simulink model "MPC_framework"  (Simulink 6.4)
settings: Solver=FixedStepDiscrete  StartTime=0.0  StopTime=10.0  FixedStep=0.01  RelTol=1e-3
PreLoadFcn:
  | RTWConfigurationCB('preloadfcn', bdroot);
InitFcn:
  | % START RTW CONFIGURATION CODE %
  | RTWConfigurationCB('rtw_target_initfcn',gcs);
  | % END RTW CONFIGURATION CODE %
values from neighbouring files (symbols this model uses):
  a1 = 1000    [param_list.m]
  a2 = 750    [param_list.m]
  increments_per_half_turn = uint32(hex2dec('400000'))    [param_list.m]
  init_1_message = uint8(1)    [param-list.m]    (also in param_list.m)
  init_2_message = uint8(2)    [param-list.m]    (also in param_list.m)
  init_ack_async_message = uint8(21)    [param-list.m]    (also in param_list.m)
  init_ack_sync_message = uint8(20)    [param-list.m]    (also in param_list.m)
  motor_negative_value = DA_max * 0.4    [param_list.m]
  motor_positive_value = DA_max * 0.6    [param_list.m]
  motor_stopped_value = DA_max / 2    [param_list.m]
libraries: canblocks x16, mpc555toucan x16, simulink x6, mpc555drivers x1
settings Model: LastModifiedBy=Developer  ProdHWDeviceType=Motorola PowerPC
settings OptimizationCC: OptimizeModelRefInitCode=on  LifeSpan=1
settings HardwareCC: ProdIntDivRoundTo=Zero  ProdEndianess=BigEndian  ProdHWDeviceType=Motorola PowerPC
settings RTWCC: SystemTargetFile=mpc555rt.tlc  TemplateMakefile=mpc555rt.tmf  Description=Embedded Target for Motorola MPC555 (real-time target)  ProcessScript=mpc555rt_make_rtw_hook
settings CodeAppCC: IgnoreCustomStorageClasses=off
settings STFCustomTargetCC: TargetFcnLib=codewarrior_tfl_tmw.mat  TargetLibSuffix=.a  TargetPreCompLibLocation=C:\MATLAB\R2006a\toolbox\rtw\targets\mpc555dk\drivers\lib\CODE_WARRIOR  GenFloatMathFcnCalls=ISO_C  CombineOutputUpdateFcns=on  IncludeERTFirstTime=on  ERTCustomFileBanners=on  SupportContinuousTime=off  SupportNonInlinedSFcns=off  SystemTargetFile=mpc555rt.tlc
settings ERTTargetCC: TargetFcnLib=codewarrior_tfl_tmw.mat  TargetPreCompLibLocation=C:\MATLAB\R2006a\toolbox\rtw\targets\mpc555dk\drivers\lib\CODE_WARRIOR  GenFloatMathFcnCalls=ISO_C  IncludeERTFirstTime=on  ERTFirstTimeCompliant=off  InlinedParameterPlacement=NonHierarchical  ERTCustomFileTemplate=example_file_process.tlc  InitialValueSource=Model
settings CustomProperty: DataType=RTWOptions_EnumType__toolbox_rtw_targets_mpc555dk_mpc555dk_mpc555rt_MPC555_OPTIMIZATION_SWITCH  Value=speed
settings EnumStrPairs: String=speed

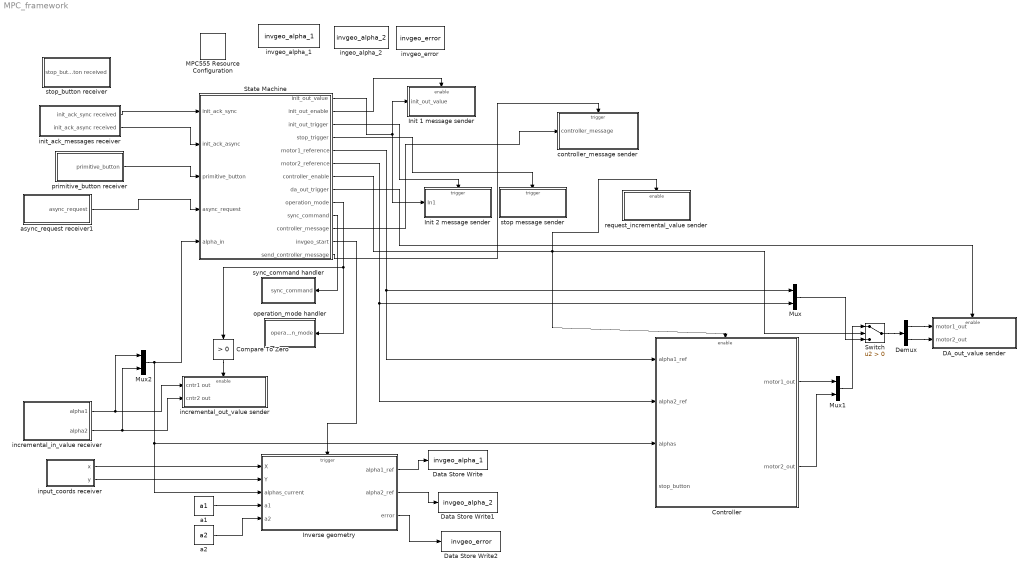
== system MPC_framework ==
  Compare To Zero : simulink/Logic and Bit Operations/Compare To Zero  Orientation=down  SystemSampleTime=-1  relop=>  LogicOutDataTypeMode=uint8  ZeroCross=off
  Controller : Subsystem
  DA_out_value sender : Subsystem  TreatAsAtomicUnit=on
  Data Store Write : DataStoreWrite  DataStoreName=invgeo_alpha_1  SampleTime=-1
  Data Store Write1 : DataStoreWrite  DataStoreName=invgeo_alpha_2  SampleTime=-1
  Data Store Write2 : DataStoreWrite  DataStoreName=invgeo_error  SampleTime=-1
  Demux : Demux  Outputs=2
  Init 1 message sender : Subsystem  TreatAsAtomicUnit=on
  Init 2 message sender : Subsystem  TreatAsAtomicUnit=on
  Inverse geometry : Subsystem  TreatAsAtomicUnit=on
  MPC555 Resource Configuration : mpc555drivers/MPC555 Resource Configuration  Tag=RTW CONFIGURATION BLOCK  Priority=-100000  SystemSampleTime=-1  oldParentName=MPC_framework  oldBlockName=|
      | MPC_framework/MPC555
      | Resource
      | Configuration
  Mux : Mux  Inputs=2
  Mux1 : Mux  Inputs=2
  Mux2 : Mux  Inputs=2
  State Machine : Stateflow chart
  Switch : Switch  Criteria=u2 > Threshold
  a1 : Constant  Value=a1  OutDataType=sfix(16)  ConRadixGroup=Use specified scaling  OutScaling=2^0  SampleTime=inf  FramePeriod=inf
  a2 : Constant  Value=a2  OutDataType=sfix(16)  ConRadixGroup=Use specified scaling  OutScaling=2^0  SampleTime=inf  FramePeriod=inf
  async_request receiver1 : Subsystem
  controller_message sender : Subsystem  TreatAsAtomicUnit=on
  incremental_in_value receiver : Subsystem
  incremental_out_value sender : Subsystem  TreatAsAtomicUnit=on
  ingeo_alpha_2 : DataStoreMemory  DataStoreName=invgeo_alpha_2  ReadBeforeWriteMsg=error  WriteAfterWriteMsg=error  WriteAfterReadMsg=error  InitialValue=0  DataType=double
  init_ack_messages receiver : Subsystem
  input_coords receiver : Subsystem
  invgeo_alpha_1 : DataStoreMemory  DataStoreName=invgeo_alpha_1  ReadBeforeWriteMsg=error  WriteAfterWriteMsg=error  WriteAfterReadMsg=error  InitialValue=0  DataType=double
  invgeo_error : DataStoreMemory  DataStoreName=invgeo_error  ReadBeforeWriteMsg=error  WriteAfterWriteMsg=error  WriteAfterReadMsg=error  InitialValue=0  DataType=uint8
  operation_mode handler : Subsystem  Orientation=left
  primitive_button receiver : Subsystem
  request_incremental_value sender : Subsystem  TreatAsAtomicUnit=on
  stop message sender : Subsystem  TreatAsAtomicUnit=on
  stop_button receiver : Subsystem
  sync_command handler : Subsystem  Orientation=left
  wires:
  State Machine/1(init_out_value) -> Init 2 message sender/1(In1), Init 1 message sender/1(init_out_value)
  State Machine/2(init_out_enable) -> Init 1 message sender/Enable
  init_ack_messages receiver/1(init_ack_sync received) -> State Machine/1(init_ack_sync)
  init_ack_messages receiver/2(init_ack_async received) -> State Machine/2(init_ack_async)
  State Machine/3(init_out_trigger) -> Init 2 message sender/Trigger
  State Machine/4(stop_trigger) -> stop message sender/Trigger
  primitive_button receiver/1(primitive_button) -> State Machine/3(primitive_button)
  State Machine/7(controller_enable) -> Switch/2, request_incremental_value sender/Enable, Controller/Enable
  State Machine/5(motor1_reference) -> Controller/1(alpha1_ref), Mux/1
  State Machine/6(motor2_reference) -> Controller/2(alpha2_ref), Mux/2
  incremental_in_value receiver/2(alpha2) -> incremental_out_value sender/2(cntr2 out), Mux2/2
  Controller/1(motor1_out) -> Mux1/1
  Controller/2(motor2_out) -> Mux1/2
  Mux1/1 -> Switch/1
  Mux/1 -> Switch/3
  Switch/1 -> Demux/1
  Demux/1 -> DA_out_value sender/1(motor1_out)
  Demux/2 -> DA_out_value sender/2(motor2_out)
  State Machine/8(da_out_trigger) -> DA_out_value sender/Enable
  State Machine/9(operation_mode) -> Compare To Zero/1, operation_mode handler/1(operation_mode)
  async_request receiver1/1(async_request) -> State Machine/4(async_request)
  Compare To Zero/1 -> incremental_out_value sender/Enable
  State Machine/10(sync_command) -> sync_command handler/1(sync_command)
  incremental_in_value receiver/1(alpha1) -> incremental_out_value sender/1(cntr1 out), Mux2/1
  Mux2/1 -> State Machine/5(alpha_in), Controller/3(alphas), Inverse geometry/3(alphas_current)
  a1/1 -> Inverse geometry/4(a1)
  a2/1 -> Inverse geometry/5(a2)
  State Machine/12(invgeo_start) -> Inverse geometry/Trigger
  State Machine/11(controller_message) -> controller_message sender/1(controller_message)
  State Machine/13(send_controller_message) -> controller_message sender/Trigger
  input_coords receiver/1(x) -> Inverse geometry/1(X)
  input_coords receiver/2(y) -> Inverse geometry/2(Y)
  Inverse geometry/1(alpha1_ref) -> Data Store Write/1
  Inverse geometry/2(alpha2_ref) -> Data Store Write1/1
  Inverse geometry/3(error) -> Data Store Write2/1

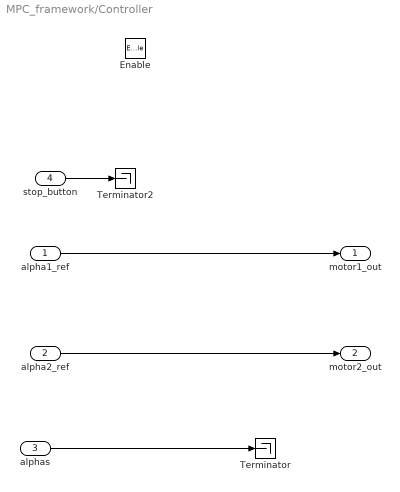
== system MPC_framework/Controller ==
  alpha1_ref : Inport
  alpha2_ref : Inport  Port=2
  alphas : Inport  Port=3
  stop_button : Inport  Port=4
  Enable : EnablePort
  Terminator : Terminator
  Terminator2 : Terminator
  motor1_out : Outport
  motor2_out : Outport  Port=2
  wires:
  alphas/1 -> Terminator/1
  alpha1_ref/1 -> motor1_out/1
  alpha2_ref/1 -> motor2_out/1
  stop_button/1 -> Terminator2/1

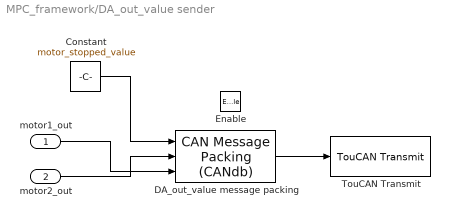
== system MPC_framework/DA_out_value sender ==
  motor1_out : Inport
  motor2_out : Inport  Port=2
  Enable : EnablePort
  Constant : Constant  Value=motor_stopped_value  OutDataType=sfix(16)  ConRadixGroup=Use specified scaling  OutScaling=2^0  SampleTime=inf  FramePeriod=inf
  DA_out_value message packing : canblocks/CAN Message Packing (CANdb)
  TouCAN Transmit : mpc555toucan/TouCAN Transmit  SystemSampleTime=-1  module=A  tx_mode=Queued transmission with shared buffer  fifo_queue_length=8  bufferids=0  buffers_used=0, 1, 2  t=-1  enablePassThru=off
  wires:
  DA_out_value message packing/1 -> TouCAN Transmit/1
  motor1_out/1 -> DA_out_value message packing/3
  motor2_out/1 -> DA_out_value message packing/2
  Constant/1 -> DA_out_value message packing/1

== system MPC_framework/Init 1 message sender ==
  init_out_value : Inport
  Enable : EnablePort
  TouCAN Transmit : mpc555toucan/TouCAN Transmit  SystemSampleTime=-1  module=A  tx_mode=Queued transmission with shared buffer  fifo_queue_length=8  bufferids=0  buffers_used=0, 1, 2  t=init_1_message_frequency  enablePassThru=off
  init message packing : canblocks/CAN Message Packing (CANdb)
  wires:
  init_out_value/1 -> init message packing/1
  init message packing/1 -> TouCAN Transmit/1

== system MPC_framework/Init 2 message sender ==
  In1 : Inport
  Trigger : TriggerPort
  TouCAN Transmit : mpc555toucan/TouCAN Transmit  SystemSampleTime=-1  module=A  tx_mode=Queued transmission with shared buffer  fifo_queue_length=8  bufferids=0  buffers_used=0, 1, 2  t=-1  enablePassThru=off
  init message packing : canblocks/CAN Message Packing (CANdb)
  wires:
  In1/1 -> init message packing/1
  init message packing/1 -> TouCAN Transmit/1

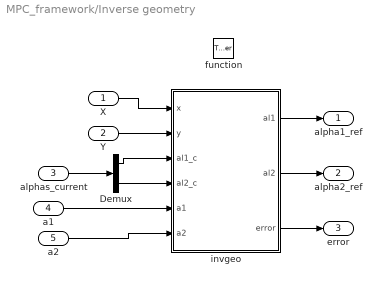
== system MPC_framework/Inverse geometry ==
  X : Inport
  Y : Inport  Port=2
  alphas_current : Inport  Port=3
  a1 : Inport  Port=4
  a2 : Inport  Port=5
  function : TriggerPort  TriggerType=function-call
  Demux : Demux  Outputs=2
  invgeo : Stateflow chart
  alpha1_ref : Outport
  alpha2_ref : Outport  Port=2
  error : Outport  Port=3
  wires:
  X/1 -> invgeo/1(x)
  Y/1 -> invgeo/2(y)
  alphas_current/1 -> Demux/1
  Demux/1 -> invgeo/3(al1_c)
  Demux/2 -> invgeo/4(al2_c)
  a1/1 -> invgeo/5(a1)
  a2/1 -> invgeo/6(a2)
  invgeo/1(al1) -> alpha1_ref/1
  invgeo/2(al2) -> alpha2_ref/1
  invgeo/3(error) -> error/1

== system MPC_framework/async_request receiver1 ==
  async_request message receive : mpc555toucan/TouCAN Receive  SystemSampleTime=-1  module=A  ids=hex2dec('0C')  notification_type=Function Call Outport  auto_select_buffer=on  bufferids=3  use_queue=off  queue_length=3  message_type=Standard (11-bit identifier)  t=-1
  async_request message unpacking : Subsystem  TreatAsAtomicUnit=on
      settings: OpenFcn=open_system(gcb, 'force');
      mask Type: CAN Message Unpacking (CANdb)
      mask Description: CAN Message Unpacking (CANdb) Function-Call Subsystem Template
      mask Help: helpview([docroot '/toolbox/can_blocks/can_blocks.map'], 'template_CANdb_msg_unpack');
  async_request : Outport
  wires:
  async_request message receive/1 -> async_request message unpacking/Trigger
  async_request message receive/2 -> async_request message unpacking/1(Msg)
  async_request message unpacking/1(async_request) -> async_request/1

== system MPC_framework/controller_message sender ==
  controller_message : Inport
  function : TriggerPort  TriggerType=function-call
  TouCAN Transmit : mpc555toucan/TouCAN Transmit  SystemSampleTime=-1  module=A  tx_mode=Queued transmission with shared buffer  fifo_queue_length=8  bufferids=0  buffers_used=0, 1, 2  t=-1  enablePassThru=off
  controller_message packing : canblocks/CAN Message Packing (CANdb)
  wires:
  controller_message packing/1 -> TouCAN Transmit/1
  controller_message/1 -> controller_message packing/1

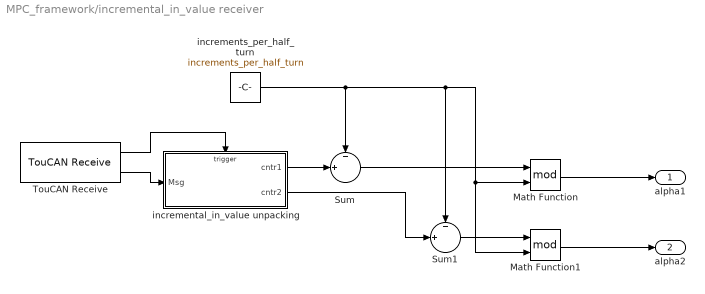
== system MPC_framework/incremental_in_value receiver ==
  Math Function : Math  Operator=mod  SaturateOnIntegerOverflow=on
  Math Function1 : Math  Operator=mod  SaturateOnIntegerOverflow=on
  Sum : Sum  Inputs=-|+||
  Sum1 : Sum  Inputs=-|+||
  TouCAN Receive : mpc555toucan/TouCAN Receive  SystemSampleTime=-1  module=A  ids=hex2dec('07')  notification_type=Function Call Outport  auto_select_buffer=on  bufferids=4  use_queue=off  queue_length=3  message_type=Standard (11-bit identifier)  t=-1
  incremental_in_value unpacking : Subsystem  TreatAsAtomicUnit=on
      settings: OpenFcn=open_system(gcb, 'force');
      mask Type: CAN Message Unpacking (CANdb)
      mask Description: CAN Message Unpacking (CANdb) Function-Call Subsystem Template
      mask Help: helpview([docroot '/toolbox/can_blocks/can_blocks.map'], 'template_CANdb_msg_unpack');
  increments_per_half_turn : Constant  Value=increments_per_half_turn  OutDataTypeMode=double  OutDataType=sfix(16)  ConRadixGroup=Use specified scaling  OutScaling=2^0  SampleTime=inf  FramePeriod=inf
  alpha1 : Outport
  alpha2 : Outport  Port=2
  wires:
  TouCAN Receive/2 -> incremental_in_value unpacking/1(Msg)
  TouCAN Receive/1 -> incremental_in_value unpacking/Trigger
  incremental_in_value unpacking/1(cntr1) -> Sum/2
  incremental_in_value unpacking/2(cntr2) -> Sum1/2
  increments_per_half_turn/1 -> Sum/1, Sum1/1, Math Function/2, Math Function1/2
  Sum/1 -> Math Function/1
  Sum1/1 -> Math Function1/1
  Math Function/1 -> alpha1/1
  Math Function1/1 -> alpha2/1

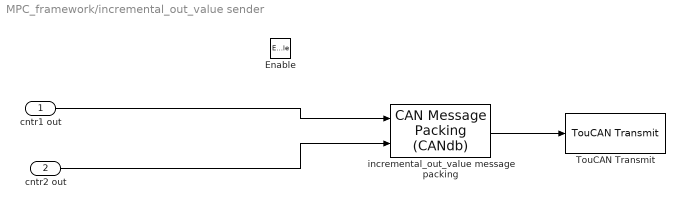
== system MPC_framework/incremental_out_value sender ==
  cntr1 out : Inport
  cntr2 out : Inport  Port=2
  Enable : EnablePort
  TouCAN Transmit : mpc555toucan/TouCAN Transmit  SystemSampleTime=-1  module=A  tx_mode=Queued transmission with shared buffer  fifo_queue_length=8  bufferids=0  buffers_used=0, 1, 2  t=-1  enablePassThru=off
  incremental_out_value message packing : canblocks/CAN Message Packing (CANdb)
  wires:
  incremental_out_value message packing/1 -> TouCAN Transmit/1
  cntr1 out/1 -> incremental_out_value message packing/1
  cntr2 out/1 -> incremental_out_value message packing/2

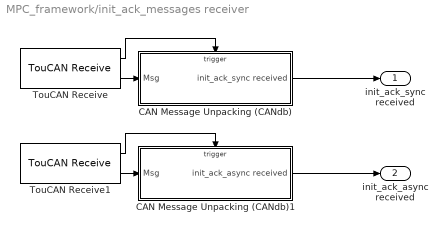
== system MPC_framework/init_ack_messages receiver ==
  CAN Message Unpacking (CANdb) : Subsystem  TreatAsAtomicUnit=on
      settings: OpenFcn=open_system(gcb, 'force');
      mask Type: CAN Message Unpacking (CANdb)
      mask Description: CAN Message Unpacking (CANdb) Function-Call Subsystem Template
      mask Help: helpview([docroot '/toolbox/can_blocks/can_blocks.map'], 'template_CANdb_msg_unpack');
  CAN Message Unpacking (CANdb)1 : Subsystem  TreatAsAtomicUnit=on
      settings: OpenFcn=open_system(gcb, 'force');
      mask Type: CAN Message Unpacking (CANdb)
      mask Description: CAN Message Unpacking (CANdb) Function-Call Subsystem Template
      mask Help: helpview([docroot '/toolbox/can_blocks/can_blocks.map'], 'template_CANdb_msg_unpack');
  TouCAN Receive : mpc555toucan/TouCAN Receive  SystemSampleTime=-1  module=A  ids=hex2dec('02')  notification_type=Function Call Outport  auto_select_buffer=on  bufferids=5  use_queue=off  queue_length=3  message_type=Standard (11-bit identifier)  t=-1
  TouCAN Receive1 : mpc555toucan/TouCAN Receive  SystemSampleTime=-1  module=A  ids=hex2dec('03')  notification_type=Function Call Outport  auto_select_buffer=on  bufferids=6  use_queue=off  queue_length=3  message_type=Standard (11-bit identifier)  t=-1
  init_ack_sync received : Outport
  init_ack_async received : Outport  Port=2
  wires:
  TouCAN Receive/1 -> CAN Message Unpacking (CANdb)/Trigger
  TouCAN Receive/2 -> CAN Message Unpacking (CANdb)/1(Msg)
  CAN Message Unpacking (CANdb)/1(init_ack_sync received) -> init_ack_sync received/1
  TouCAN Receive1/1 -> CAN Message Unpacking (CANdb)1/Trigger
  TouCAN Receive1/2 -> CAN Message Unpacking (CANdb)1/1(Msg)
  CAN Message Unpacking (CANdb)1/1(init_ack_async received) -> init_ack_async received/1

== system MPC_framework/input_coords receiver ==
  async_request message receive : mpc555toucan/TouCAN Receive  SystemSampleTime=-1  module=A  ids=hex2dec('10')  notification_type=Function Call Outport  auto_select_buffer=on  bufferids=7  use_queue=off  queue_length=3  message_type=Standard (11-bit identifier)  t=-1
  input_coords message unpacking : Subsystem  TreatAsAtomicUnit=on
      settings: OpenFcn=open_system(gcb, 'force');
      mask Type: CAN Message Unpacking (CANdb)
      mask Description: CAN Message Unpacking (CANdb) Function-Call Subsystem Template
      mask Help: helpview([docroot '/toolbox/can_blocks/can_blocks.map'], 'template_CANdb_msg_unpack');
  x : Outport
  y : Outport  Port=2
  wires:
  input_coords message unpacking/1(x) -> x/1
  async_request message receive/2 -> input_coords message unpacking/1(Msg)
  async_request message receive/1 -> input_coords message unpacking/Trigger
  input_coords message unpacking/2(y) -> y/1

== system MPC_framework/operation_mode handler ==
  operation_mode : Inport
  Detect Change : simulink/Logic and Bit Operations/Detect Change  SystemSampleTime=-1  vinit=0
  operation_mode_changed sender : Subsystem  TreatAsAtomicUnit=on
  wires:
  Detect Change/1 -> operation_mode_changed sender/Trigger
  operation_mode/1 -> operation_mode_changed sender/1(operation_mode), Detect Change/1

== system MPC_framework/primitive_button receiver ==
  primitive_button message receive : mpc555toucan/TouCAN Receive  SystemSampleTime=-1  module=A  ids=hex2dec('08')  notification_type=Function Call Outport  auto_select_buffer=on  bufferids=8  use_queue=off  queue_length=3  message_type=Standard (11-bit identifier)  t=-1
  primitive_button message unpacking : Subsystem  TreatAsAtomicUnit=on
      settings: OpenFcn=open_system(gcb, 'force');
      mask Type: CAN Message Unpacking (CANdb)
      mask Description: CAN Message Unpacking (CANdb) Function-Call Subsystem Template
      mask Help: helpview([docroot '/toolbox/can_blocks/can_blocks.map'], 'template_CANdb_msg_unpack');
  primitive_button : Outport
  wires:
  primitive_button message unpacking/1("primitive_button ") -> primitive_button/1
  primitive_button message receive/2 -> primitive_button message unpacking/1(Msg)
  primitive_button message receive/1 -> primitive_button message unpacking/Trigger

== system MPC_framework/request_incremental_value sender ==
  Enable : EnablePort
  Constant : Constant  Value=1  OutDataTypeMode=uint8  OutDataType=sfix(16)  ConRadixGroup=Use specified scaling  OutScaling=2^0  SampleTime=0.1  FramePeriod=inf
  TouCAN Transmit : mpc555toucan/TouCAN Transmit  SystemSampleTime=-1  module=A  tx_mode=Queued transmission with shared buffer  fifo_queue_length=8  bufferids=0  buffers_used=0, 1, 2  t=-1  enablePassThru=off
  request_incremental_value message packing : canblocks/CAN Message Packing (CANdb)
  wires:
  Constant/1 -> request_incremental_value message packing/1
  request_incremental_value message packing/1 -> TouCAN Transmit/1

== system MPC_framework/stop message sender ==
  Trigger : TriggerPort
  Constant : Constant  Value=1  OutDataTypeMode=uint8  OutDataType=sfix(16)  ConRadixGroup=Use specified scaling  OutScaling=2^0  SampleTime=inf  FramePeriod=inf
  TouCAN Transmit : mpc555toucan/TouCAN Transmit  SystemSampleTime=-1  module=A  tx_mode=Queued transmission with shared buffer  fifo_queue_length=8  bufferids=0  buffers_used=0, 1, 2  t=-1  enablePassThru=off
  stop message packing : canblocks/CAN Message Packing (CANdb)
  wires:
  stop message packing/1 -> TouCAN Transmit/1
  Constant/1 -> stop message packing/1

== system MPC_framework/stop_button receiver ==
  TouCAN Receive : mpc555toucan/TouCAN Receive  SystemSampleTime=-1  module=A  ids=hex2dec('04')  notification_type=Function Call Outport  auto_select_buffer=on  bufferids=9  use_queue=off  queue_length=3  message_type=Standard (11-bit identifier)  t=-1
  stop_button message packing : Subsystem  TreatAsAtomicUnit=on
      settings: OpenFcn=open_system(gcb, 'force');
      mask Type: CAN Message Unpacking (CANdb)
      mask Description: CAN Message Unpacking (CANdb) Function-Call Subsystem Template
      mask Help: helpview([docroot '/toolbox/can_blocks/can_blocks.map'], 'template_CANdb_msg_unpack');
  stop_button received : Outport
  wires:
  TouCAN Receive/1 -> stop_button message packing/Trigger
  TouCAN Receive/2 -> stop_button message packing/1(Msg)
  stop_button message packing/1(stop_button received) -> stop_button received/1

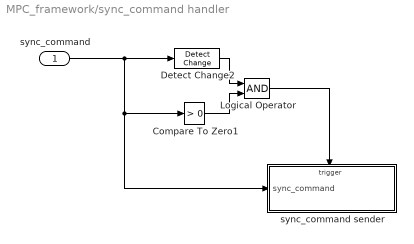
== system MPC_framework/sync_command handler ==
  sync_command : Inport
  Compare To Zero1 : simulink/Logic and Bit Operations/Compare To Zero  SystemSampleTime=-1  relop=>  LogicOutDataTypeMode=uint8  ZeroCross=off
  Detect Change2 : simulink/Logic and Bit Operations/Detect Change  SystemSampleTime=-1  vinit=0
  Logical Operator : Logic  AllPortsSameDT=off  OutDataTypeMode=Boolean
  sync_command sender : Subsystem  TreatAsAtomicUnit=on
  wires:
  Detect Change2/1 -> Logical Operator/1
  Compare To Zero1/1 -> Logical Operator/2
  Logical Operator/1 -> sync_command sender/Trigger
  sync_command/1 -> Detect Change2/1, Compare To Zero1/1, sync_command sender/1(sync_command)

== system MPC_framework/async_request receiver1/async_request message unpacking ==
  note: Add any blocks to this subsystem that need to be
      | executed each time a message is received.
  Msg : Inport
  f : TriggerPort  TriggerType=function-call
  CAN Message Unpacking (CANdb) : canblocks/CAN Message Unpacking (CANdb)/CAN Message Unpacking (CANdb)
  async_request : Outport
  wires:
  Msg/1 -> CAN Message Unpacking (CANdb)/1
  CAN Message Unpacking (CANdb)/1 -> async_request/1

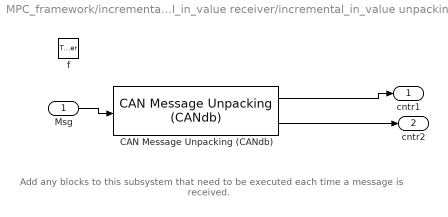
== system MPC_framework/incremental_in_value receiver/incremental_in_value unpacking ==
  note: Add any blocks to this subsystem that need to be
      | executed each time a message is received.
  Msg : Inport
  f : TriggerPort  TriggerType=function-call
  CAN Message Unpacking (CANdb) : canblocks/CAN Message Unpacking (CANdb)/CAN Message Unpacking (CANdb)
  cntr1 : Outport
  cntr2 : Outport  Port=2
  wires:
  CAN Message Unpacking (CANdb)/1 -> cntr1/1
  Msg/1 -> CAN Message Unpacking (CANdb)/1
  CAN Message Unpacking (CANdb)/2 -> cntr2/1

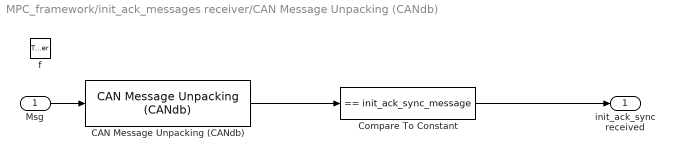
== system MPC_framework/init_ack_messages receiver/CAN Message Unpacking (CANdb) ==
  Msg : Inport
  f : TriggerPort  TriggerType=function-call
  CAN Message Unpacking (CANdb) : canblocks/CAN Message Unpacking (CANdb)/CAN Message Unpacking (CANdb)
  Compare To Constant : simulink/Logic and Bit Operations/Compare To Constant  SystemSampleTime=-1  relop===  const=init_ack_sync_message  LogicOutDataTypeMode=uint8  ZeroCross=off
  init_ack_sync received : Outport
  wires:
  Msg/1 -> CAN Message Unpacking (CANdb)/1
  CAN Message Unpacking (CANdb)/1 -> Compare To Constant/1
  Compare To Constant/1 -> init_ack_sync received/1

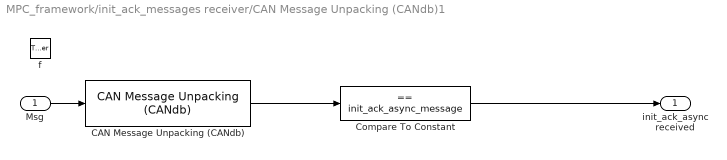
== system MPC_framework/init_ack_messages receiver/CAN Message Unpacking (CANdb)1 ==
  Msg : Inport
  f : TriggerPort  TriggerType=function-call
  CAN Message Unpacking (CANdb) : canblocks/CAN Message Unpacking (CANdb)/CAN Message Unpacking (CANdb)
  Compare To Constant : simulink/Logic and Bit Operations/Compare To Constant  SystemSampleTime=-1  relop===  const=init_ack_async_message  LogicOutDataTypeMode=uint8  ZeroCross=off
  init_ack_async received : Outport
  wires:
  Compare To Constant/1 -> init_ack_async received/1
  CAN Message Unpacking (CANdb)/1 -> Compare To Constant/1
  Msg/1 -> CAN Message Unpacking (CANdb)/1

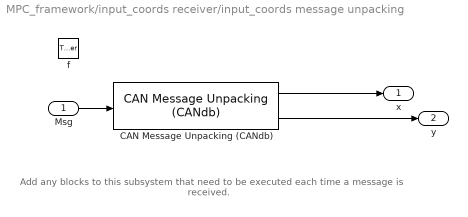
== system MPC_framework/input_coords receiver/input_coords message unpacking ==
  note: Add any blocks to this subsystem that need to be
      | executed each time a message is received.
  Msg : Inport
  f : TriggerPort  TriggerType=function-call
  CAN Message Unpacking (CANdb) : canblocks/CAN Message Unpacking (CANdb)/CAN Message Unpacking (CANdb)
  x : Outport
  y : Outport  Port=2
  wires:
  CAN Message Unpacking (CANdb)/1 -> x/1
  Msg/1 -> CAN Message Unpacking (CANdb)/1
  CAN Message Unpacking (CANdb)/2 -> y/1

== system MPC_framework/operation_mode handler/operation_mode_changed sender ==
  operation_mode : Inport
  Trigger : TriggerPort
  TouCAN Transmit : mpc555toucan/TouCAN Transmit  SystemSampleTime=-1  module=A  tx_mode=Queued transmission with shared buffer  fifo_queue_length=8  bufferids=0  buffers_used=0, 1, 2  t=-1  enablePassThru=off
  operation_mode_changed message packing : canblocks/CAN Message Packing (CANdb)
  wires:
  operation_mode_changed message packing/1 -> TouCAN Transmit/1
  operation_mode/1 -> operation_mode_changed message packing/1

== system MPC_framework/primitive_button receiver/primitive_button message unpacking ==
  note: Add any blocks to this subsystem that need to be
      | executed each time a message is received.
  Msg : Inport
  f : TriggerPort  TriggerType=function-call
  CAN Message Unpacking (CANdb) : canblocks/CAN Message Unpacking (CANdb)/CAN Message Unpacking (CANdb)
  "primitive_button " : Outport
  wires:
  CAN Message Unpacking (CANdb)/1 -> "primitive_button "/1
  Msg/1 -> CAN Message Unpacking (CANdb)/1

== system MPC_framework/stop_button receiver/stop_button message packing ==
  note: Add any blocks to this subsystem that need to be
      | executed each time a message is received.
  Msg : Inport
  f : TriggerPort  TriggerType=function-call
  CAN Message Unpacking (CANdb) : canblocks/CAN Message Unpacking (CANdb)/CAN Message Unpacking (CANdb)
  stop_button received : Outport
  wires:
  Msg/1 -> CAN Message Unpacking (CANdb)/1
  CAN Message Unpacking (CANdb)/1 -> stop_button received/1

== system MPC_framework/sync_command handler/sync_command sender ==
  sync_command : Inport
  Trigger : TriggerPort
  TouCAN Transmit : mpc555toucan/TouCAN Transmit  SystemSampleTime=-1  module=A  tx_mode=Queued transmission with shared buffer  fifo_queue_length=8  bufferids=0  buffers_used=0, 1, 2  t=-1  enablePassThru=off
  sync_command message packing : canblocks/CAN Message Packing (CANdb)
  wires:
  sync_command/1 -> sync_command message packing/1
  sync_command message packing/1 -> TouCAN Transmit/1

== stateflow chart State Machine ==
  settings: updateMethod=DISCRETE  sampleTime=0.01  executeAtInitialization=1
  state INIT
    entry: init_out_value=init_1_message;
    init_out_enable=1;
  state INIT_ACK
    entry: init_out_enable=0;
    init_out_value=init_2_message;
    init_out_trigger=1;
  state OPERATION
    entry: operation_mode=255;
    state PRIMITIVE
      entry: operation_mode=1;
      during: controller_enable=0;
      state STOPPED
        entry: motor1_reference=motor_stopped_value;
        motor2_reference=motor_stopped_value;
        da_out_trigger=1;
        during: da_out_trigger=0;
        exit: stop_trigger=0;
      state MOVING
        state SEGMENT_1 [parallel]
          settings: executionOrder=1
          state POSITIVE_MOV
            entry:
            motor1_reference=motor_positive_value;
            da_out_trigger=1;
            during:
            da_out_trigger=0;
          state NEGATIVE_MOV
            entry:
            motor1_reference=motor_negative_value;
            da_out_trigger=1;
            during:
            da_out_trigger=0;
          (default) -> OPERATION.PRIMITIVE.MOVING.SEGMENT_1.POSITIVE_MOV
        state SEGMENT_2 [parallel]
          settings: executionOrder=2
          state POSITIVE_MOV
            entry:
            motor2_reference=motor_positive_value;
            da_out_trigger=1;
            during:
            da_out_trigger=0;
          state NEGATIVE_MOV
            entry:
            motor2_reference=motor_negative_value;
            da_out_trigger=1;
            during:
            da_out_trigger=0;
          (default) -> OPERATION.PRIMITIVE.MOVING.SEGMENT_2.POSITIVE_MOV
      (default) -> STOPPED
      MOVING -> STOPPED : [primitive_button==5]
      STOPPED -> OPERATION.PRIMITIVE.MOVING.SEGMENT_1.POSITIVE_MOV [order 4] : [primitive_button==1]
      STOPPED -> OPERATION.PRIMITIVE.MOVING.SEGMENT_1.NEGATIVE_MOV [order 2] : [primitive_button==3]
      STOPPED -> OPERATION.PRIMITIVE.MOVING.SEGMENT_2.POSITIVE_MOV [order 3] : [primitive_button==2]
      STOPPED -> OPERATION.PRIMITIVE.MOVING.SEGMENT_2.NEGATIVE_MOV [order 1] : [primitive_button==4]
    state CONTROLLER
      entry: operation_mode=2;
      alpha1_ref=alpha_in[0];
      alpha2_ref=alpha_in[1];
      invgeo_error=255;
      state HOLD
        entry:
        during: controller_enable=1;
        motor1_reference=alpha1_ref;
        motor2_reference=alpha2_ref;
      state TRAJECTORY
      (default) -> HOLD
      HOLD -> HOLD [order 3] : [async_request==10]{invgeo_start}
      HOLD -> (junction 20) [order 1] : [invgeo_error==1]{controller_message=2}
      (junction 20) -> HOLD : /send_controller_message
      HOLD -> (junction 20) [order 2] : [invgeo_error==0]{controller_message=2}
    state CONFIG
      entry: operation_mode=3;
      during: controller_enable=0;
      sync_command=0;
    state BLUETOOTH
      entry: operation_mode=4;
      during: controller_enable=0;
    (default) -> PRIMITIVE
    PRIMITIVE -> CONTROLLER [order 1] : [async_request==2]
    CONTROLLER -> PRIMITIVE [order 1] : [async_request==1]
    PRIMITIVE -> CONFIG [order 3] : [async_request==6]
    CONTROLLER -> CONFIG [order 3] : [async_request==6]
    CONFIG -> PRIMITIVE [order 1] : [async_request==1]
    CONFIG -> CONTROLLER [order 2] : [async_request==2]
    CONFIG -> CONFIG [order 7] : [async_request==3]{sync_command=1}
    CONFIG -> CONFIG [order 6] : [async_request==4]{sync_command=2}
    CONFIG -> CONFIG [order 5] : [async_request==5]{sync_command=3}
    CONFIG -> CONFIG [order 4] : [async_request==7]{sync_command=4}
    CONTROLLER -> BLUETOOTH [order 2] : [async_request==8]
    PRIMITIVE -> BLUETOOTH [order 2] : [async_request==8]
    CONFIG -> BLUETOOTH [order 3] : [async_request==8]
    BLUETOOTH -> CONFIG [order 3] : [async_request==6]
    BLUETOOTH -> CONTROLLER [order 2] : [async_request==2]
    BLUETOOTH -> PRIMITIVE [order 1] : [async_request==1]
  (default) -> INIT
  INIT -> INIT_ACK : [init_ack_sync==1 && init_ack_async==1]
  INIT_ACK -> OPERATION
  data: init_out_value output uint8 =0; init_out_enable output uint8 =0; init_ack_sync input uint8; init_ack_async input uint8; init_out_trigger output uint8 =0; stop_trigger output uint8 =0; primitive_button input uint8 =0; motor1_reference output double =hex2dec('8000'); motor2_reference output double =hex2dec('8000'); motor_stopped_value parameter uint16 =hex2dec('8000'); controller_enable output uint8 =0; init_1_message parameter uint8 =init_1_message; init_2_message parameter uint8 =init_2_message; motor_positive_value parameter uint16; motor_negative_value parameter uint16; da_out_trigger output double =0; async_request input double; operation_mode output uint8 =255; sync_command output uint8 =0; alpha1_ref local double; alpha2_ref local double; alpha_in input double size=[1 2]; controller_message output uint8; invgeo_error data_store_memory double
  events: invgeo_start output FUNCTION_CALL_EVENT; send_controller_message output FUNCTION_CALL_EVENT

== matlab function Inverse geometry/invgeo ==
  data: x input inherited; y input inherited; al1_c input inherited; al2_c input inherited; a1 input inherited; a2 input inherited; al1 output inherited; al2 output inherited; error output inherited
function [al1, al2, error] = invgeo(x, y, al1_c, al2_c, a1, a2)
    
    d = x^2 + y^2;
    if ((d > (a1^2 + a2^2)) | (d < (a1 - a2)))
        al1 = al1_c;
        al2 = al2_c;
        error = uint8(1);
        return;
    end
    
    cos_al2 = (x^2 + y^2 - a1^2 - a2^2) / (2 * a1 * a2);
    D = a1 + a2 * cos_al2;
    
    sin_al1_p = (D * y + x * sqrt(x^2 + y^2 - D^2)) / (x^2 + y^2);
    sin_al1_n = (D * y - x * sqrt(x^2 + y^2 - D^2)) / (x^2 + y^2);
    
    cos_al1_p = (D * x + y * sqrt(x^2 + y^2 - D^2)) / (x^2 + y^2);
    cos_al1_n = (D * x - y * sqrt(x^2 + y^2 - D^2)) / (x^2 + y^2);
    
    al1_1 = atan2(sin_al1_p, cos_al1_n);
    
    al1_2 = atan2(sin_al1_n, cos_al1_p);
    
    al2_p = acos(cos_al2);
    al2_n = -al2_p; 
    
    if ( x == (a1 * cos_al1_n + a2 * cos(al1_1 + al2_p)))
        al2_1 = al2_p;
        al2_2 = al2_n;
    else 
       al2_1 = al2_n;
       al2_2 = al2_p;
    end
    
    if (abs(al1_c - al1_1) < abs(al1_c - al1_2))
        al1 = al1_1;
        al2 = al2_1;
    else
        al1 = al1_2;
        al2 = al2_2;
    end
    
    error = uint8(0);  
end
